simulink model "rtwdemo_dowhilesl"  (Simulink 7.1)
settings: Solver=FixedStepDiscrete  StartTime=0.0  StopTime=10.0  FixedStep=.01  RelTol=1e-3
settings Model: Creator=ajayaram  LastModifiedBy=ajayaram
settings OptimizationCC: InlineParams=on  InlineInvariantSignals=on  OptimizeModelRefInitCode=on  LifeSpan=1
settings DebuggingCC: SaveWithParameterizedLinksMsg=none  StrictBusMsg=ErrorLevel1
settings RTWCC: SystemTargetFile=ert.tlc  GenCodeOnly=on  GenerateMakefile=off  TemplateMakefile=ert_default_tmf  Description=Real-Time Workshop Embedded Coder (no auto configuration)  GenerateReport=on  ProcessScript=ert_make_rtw_hook  IncludeHyperlinkInReport=on  LaunchReport=on
settings CodeAppCC: GenerateComments=off  IgnoreCustomStorageClasses=off  SimulinkBlockComments=off
settings ERTTargetCC: TargetFcnLib=ansi_tfl_tmw.mat  GenerateSampleERTMain=on  InlinedParameterPlacement=NonHierarchical  ERTCustomFileTemplate=example_file_process.tlc

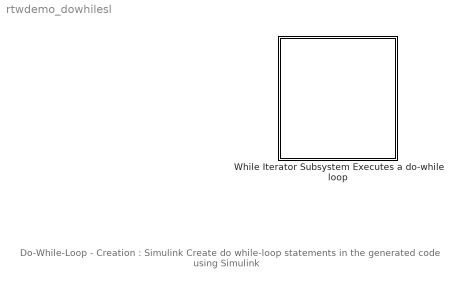
== system rtwdemo_dowhilesl ==
  note: Do-While-Loop - Creation : Simulink
      | Create do while-loop statements in the
      | generated code using Simulink
  While Iterator Subsystem Executes a do-while loop : Subsystem  TreatAsAtomicUnit=on

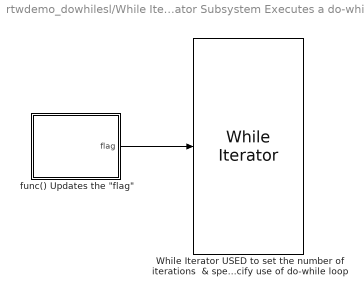
== system rtwdemo_dowhilesl/While Iterator Subsystem Executes a do-while loop ==
  While Iterator USED to set the number of iterations  & specify use of do-while loop : WhileIterator  MaxIters=100  WhileBlockType=do-while  ResetStates=reset
  "func() Updates the \"flag\"" : Subsystem  TreatAsAtomicUnit=on  RTWFcnName=func  RTWFileName=whilesl
      settings: RTWSystemCode=Function  RTWFcnNameOpts=User specified
  wires:
  "func() Updates the \"flag\""/1(flag) -> While Iterator USED to set the number of iterations  & specify use of do-while loop/1

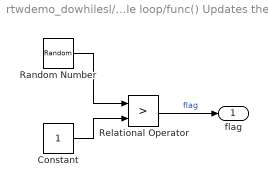
== system rtwdemo_dowhilesl/While Iterator Subsystem Executes a do-while loop/func() Updates the "flag" ==
  Constant : Constant  OutDataType=sfix(16)  OutScaling=2^0
  Random Number : RandomNumber  Variance=3
  Relational Operator : RelationalOperator  Operator=>  LogicOutDataTypeMode=boolean  OutDataTypeStr=boolean
  flag : Outport  OutDataType=sfix(16)  OutScaling=2^0
  wires:
  Relational Operator/1 -> flag/1  "flag"
  Random Number/1 -> Relational Operator/1
  Constant/1 -> Relational Operator/2
